simulink model "Quadcopter_BLDC"  (R2024a)
settings: Solver=ode45  StartTime=0.0  StopTime=5  RelTol=1e-3
settings Model: Creator=Pranav Lakshmanan  LastModifiedBy=Pranav Lakshmanan

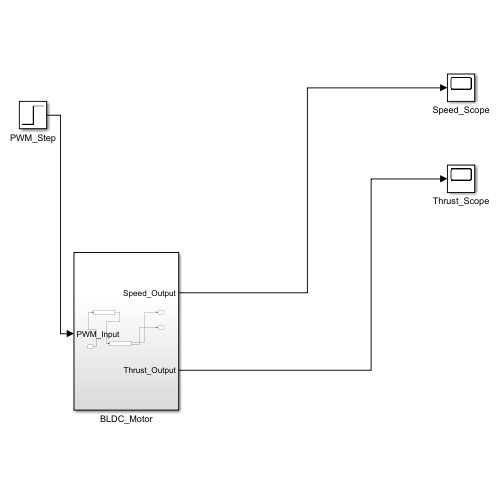
[thumbnail: Simulink's stored preview of the top-level diagram]
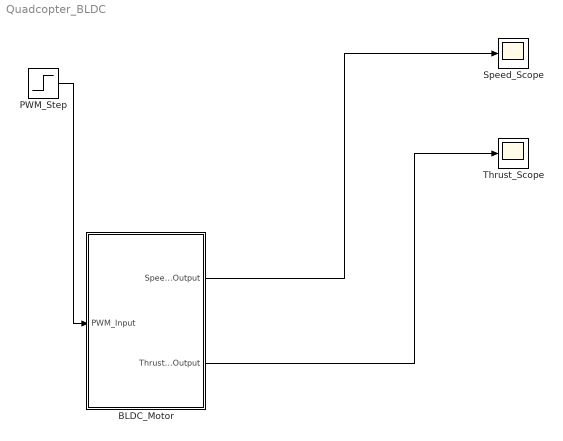
== system Quadcopter_BLDC ==
  BLDC_Motor : Subsystem
  PWM_Step : Step  Before=1000  After=2000  SampleTime=0
  Speed_Scope : Scope
  Thrust_Scope : Scope
  wires:
  BLDC_Motor/1(Speed_Output) -> Speed_Scope/1
  PWM_Step/1 -> BLDC_Motor/1(PWM_Input)
  BLDC_Motor/2(Thrust_Output) -> Thrust_Scope/1

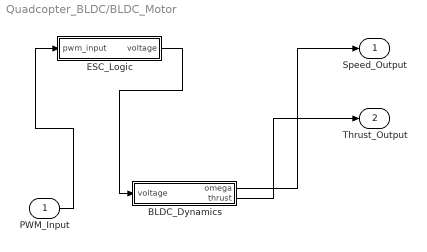
== system Quadcopter_BLDC/BLDC_Motor ==
  PWM_Input : Inport
  BLDC_Dynamics : MATLAB Function  TreatAsAtomicUnit=on
  ESC_Logic : MATLAB Function  TreatAsAtomicUnit=on
  Speed_Output : Outport
  Thrust_Output : Outport  Port=2
  wires:
  PWM_Input/1 -> ESC_Logic/1(pwm_input)
  ESC_Logic/1(voltage) -> BLDC_Dynamics/1(voltage)
  BLDC_Dynamics/1(omega) -> Speed_Output/1
  BLDC_Dynamics/2(thrust) -> Thrust_Output/1

== matlab function Quadcopter_BLDC/BLDC_Motor/ESC_Logic ==
  data: pwm_input input; voltage output
function voltage = fcn(pwm_input)
    % Convert PWM (1000-2000us) to voltage (0-12V)
    min_pwm = 1000;
    max_pwm = 2000;
    max_voltage = 12;
    
    % Normalize PWM input
    duty_cycle = (pwm_input - min_pwm)/(max_pwm - min_pwm);
    duty_cycle = max(0, min(1, duty_cycle));
    
    % Convert to voltage
    voltage = duty_cycle * max_voltage;
end

== matlab function Quadcopter_BLDC/BLDC_Motor/BLDC_Dynamics ==
  data: voltage input; omega output; thrust output
function [omega, thrust] = fcn(voltage)
    persistent curr_omega i_q;
    if isempty(curr_omega)
        curr_omega = 0;
        i_q = 0;
    end
    
    % Motor parameters
    Rs = 0.135;      % Stator resistance (Ohm)
    Ls = 0.000169;   % Stator inductance (H)
    Ke = 0.0136;     % Back-EMF constant (V/rad/s)
    Kt = 0.0136;     % Torque constant (N-m/A)
    J = 0.0000135;   % Rotor inertia (kg-m^2)
    B = 0.000000916; % Viscous friction (N-m-s/rad)
    
    Ts = 0.001; % 1kHz simulation rate
    
    % Back-EMF
    bemf = Ke * curr_omega;
    
    % Q-axis current dynamics
    di_q = (voltage - Rs*i_q - bemf)/Ls;
    i_q = i_q + di_q*Ts;
    
    % Torque calculation
    Te = Kt * i_q;
    
    % Mechanical dynamics
    domega = (Te - B*curr_omega)/J;
    curr_omega = curr_omega + domega*Ts;
    
    % Calculate thrust
    Kt_prop = 1.1e-6; % Propeller thrust coefficient
    thrust = Kt_prop * curr_omega^2;
    
    % Outputs
    omega = curr_omega;
end
